simulink library "ddm"  (R2021b)
settings: Solver=VariableStepAuto  StartTime=0.0  StopTime=10.0  RelTol=1e-3
undefined symbols (not defined in the file or in its folder): ADDM_FrTMTqDev_X_Nm, ADDM_RrTMTqDev_X_Nm, ENUM_ADASACCSTA_ERROR, ENUM_ADASACCSTA_OFF, ENUM_ADASACCSTA_STANDBY, ENUM_ALLOWMOV_ALLOWREADY, ENUM_APS, ENUM_BRKSTA_ERROR, ENUM_BRKSTA_OFF, ENUM_BRKSTA_ON, ENUM_BRKSW_INVALID, ENUM_BRKSW_OFF, ENUM_BRKSW_ON, ENUM_CHGPREACTERRSTA_OBCPRE, ENUM_DCDCFAULTSTA_ANYFAULTLV1, ENUM_DCDCFAULTSTA_ANYFAULTLV2, ENUM_DRIVETRAIN_AWD, ENUM_DRIVETRAIN_FWD, ENUM_DRIVETRAIN_RWD, ENUM_EDUDRTSTA_NORMAL, ENUM_EPBSTA_APPLIED, ENUM_EPBSTA_RELEASED, ENUM_GEARACTUALPOSN_INVALID, ENUM_GEARACTUALPOSN_P, ENUM_HVBATTREADYPRE_READY, ENUM_MCUWARN_LV0, ENUM_MCUWARN_LV1, ENUM_MCUWARN_LV2, ENUM_MCUWARN_LV3, ENUM_MCUWARN_NOERROR, ENUM_OBCFAULTSTA_ANYFAULT, ENUM_PAS_R2F2, ENUM_PDFAULT_BATTPDFAIL, ENUM_PDFAULT_DCDCDISABLE, ENUM_PDFAULT_MCUDISABLE, ENUM_PDFAULT_MCUDISCHRG, ENUM_POWERSTA_OFF, ENUM_POWERSTA_ON, ENUM_POWERSTA_READY, ENUM_POWERSTA_STANDBY, ENUM_PRESSINDI_LOW, ENUM_PUFAULT_BATTUPFAIL, ENUM_PUFAULT_DCDCENABLEFAIL, ENUM_PUFAULT_PRECHRGCHKFAIL, ENUM_PUFAULT_SAFETYCHKFAIL, ENUM_PUSTATE_COMPLETED, ENUM_PWRSTASW_OFF, ENUM_PWRSTASW_OFFA, ENUM_PWRSTASW_OFFCHVCHRG, ENUM_PWRSTASW_OFFCLVCHRG, ENUM_PWRSTASW_ON, ENUM_PWRSTASW_ONHVCHRG, ENUM_PWRSTASW_READY, ENUM_PWRSTASW_STANDBY, ENUM_SHIFTCOMMAND_P, ENUM_SHIFTERERRSTA_PBUTTONFAILURE, ENUM_VEHMALFUNLV_2ND, ENUM_VEHMALFUNLV_3RD, ENUM_VEHMALFUNLV_4TH, ENUM_VEHMALFUNLV_NORMAL ... (+459)
libraries: hcu_lib x515, simulink x3
(part 17 of 25)

== system ddm/DDM/DDM/PMM/Comm err/The CAN signal between VCU and BMS1 is discontinuous ==
  note: Test Detection Criteria
  note: Test Pass Criteria
  note: Release Condition After Decision
  note: Diagnostics and Fault Handling
  task_time_s : Inport
  VPMM_PowerSta_enum : Inport  Port=2
  VPMM_PwrStaSW_enum : Inport  Port=3
  VDDM_C3BMS1RCChk_flg : Inport  Port=4
  VDDM_C3BMS1LCCFS_flg : Inport  Port=5
  No_CAN3_BUS_OFF : Inport  Port=6
  DTC_clear_request : Inport  Port=7
  Constant1 : Constant  Value=TRUE
  Constant10 : Constant  Value=ENUM_POWERSTA_STANDBY
  Constant11 : Constant  Value=ZERO_INT
  Constant12 : Constant  Value=FALSE
  Constant13 : Constant  Value=KDDM_C3BMS1RCDTC_cnt
  Constant14 : Constant  Value=KDDM_C3BMS1RCDetTO_s
  Constant17 : Constant  Value=KDDM_C3BMS1RCDTC_cnt
  Constant29 : Constant  Value=ENUM_PWRSTASW_OFF
  Constant30 : Constant  Value=KDDM_CommErrDiagnosisOffSW_flg
  Constant31 : Constant  Value=ENUM_POWERSTA_OFF
  Constant6 : Constant  Value=KDDM_C3BMS1RCPassTO_s
  Constant7 : Constant  Value=KDDM_C3BMS1RCPassTO_s
  Constant8 : Constant  Value=FALSE
  Constant9 : Constant  Value=ENUM_PWRSTASW_OFF
  DTC_Couter1 : hcu_lib/Basic_Blocks/DTC_Couter
  DTC_Info : hcu_lib/Basic_Blocks/DTC_Info
  Delay1 : Delay  DelayLength=1
  Equal1 : RelationalOperator  Operator=~=  OutDataTypeStr=boolean  RndMeth=Simplest
  Equal5 : RelationalOperator  Operator=~=  OutDataTypeStr=boolean  RndMeth=Simplest
  Equal6 : RelationalOperator  OutDataTypeStr=boolean  RndMeth=Simplest
  Equal7 : RelationalOperator  Operator===  OutDataTypeStr=boolean  RndMeth=Simplest
  Equal8 : RelationalOperator  Operator===  OutDataTypeStr=boolean  RndMeth=Simplest
  Logical Operator10 : Logic  Operator=NOT  AllPortsSameDT=off  OutDataTypeStr=boolean
  Logical Operator11 : Logic  Inputs=3  AllPortsSameDT=off  OutDataTypeStr=boolean
  Logical Operator13 : Logic  Operator=NOT  AllPortsSameDT=off  OutDataTypeStr=boolean
  Logical Operator14 : Logic  Operator=OR  Inputs=4  AllPortsSameDT=off  OutDataTypeStr=boolean
  Logical Operator16 : Logic  AllPortsSameDT=off  OutDataTypeStr=boolean
  Logical Operator17 : Logic  Inputs=3  AllPortsSameDT=off  OutDataTypeStr=boolean
  Logical Operator20 : Logic  Operator=NOT  AllPortsSameDT=off  OutDataTypeStr=boolean
  Logical Operator22 : Logic  AllPortsSameDT=off  OutDataTypeStr=boolean
  NOT1 : Logic  Operator=NOT  AllPortsSameDT=off  OutDataTypeStr=boolean
  Relational Operator1 : RelationalOperator  Operator=>  OutDataTypeStr=boolean  RndMeth=Simplest
  Switch2 : Switch  Criteria=u2 ~= 0
  Switch8 : Switch  Criteria=u2 ~= 0
  Switch9 : Switch  Criteria=u2 ~= 0
  Terminator : Terminator
  Test Detection Criteria : hcu_lib/Basic_Blocks/Test Detection Criteria
  Timer2 : hcu_lib/Basic_Blocks/Timer
  Unit Delay1 : UnitDelay  SampleTime=-1  HasFrameUpgradeWarning=on
  VDDM_C3BMS1RCDTC_raw32 : Outport
  VDDM_C3BMS1RCCFS_flg : Outport  Port=2
  wires:
  [VDDM_C3BMS1RCCFS_flg] -> VDDM_C3BMS1RCCFS_flg/1
  DTC_Couter1/2 -> Relational Operator1/1  "VDDM_C3BMS1RCDTC_cnt"
  Constant6/1 -> Timer2/4
  DTC_Couter1/1 -> [VDDM_C3BMS1RCCFS_flg]  "VDDM_C3BMS1RCCFS_flg"
  Delay1/1 -> NOT1/1
  [VDDM_C3BMS1RCDet_flg] -> DTC_Couter1/1
  Logical Operator16/1 -> Logical Operator14/1
  Unit Delay1/1 -> Equal7/1
  Equal1/1 -> Logical Operator11/2
  [DTC_clear_request] -> Logical Operator14/2
  Constant31/1 -> Equal7/2
  Equal7/1 -> Logical Operator16/1
  Test Detection Criteria/1 -> [VDDM_C3BMS1RCDet_flg]  "VDDM_C3BMS1RCDet_flg"
  [VPMM_PowerSta_enum] -> Equal8/1
  Switch9/1 -> Test Detection Criteria/1
  Constant30/1 -> Logical Operator14/4
  Constant10/1 -> Equal8/2
  [task_time_s] -> Timer2/3
  Logical Operator14/1 -> [VDDM_C3BMS1RCCFSRls_flg]  "VDDM_C3BMS1RCCFSRls_flg"
  [VDDM_C3BMS1RCChk_flg] -> Switch8/1
  [VDDM_C3BMS1RCCFS_flg] -> Delay1/1
  Constant13/1 -> Test Detection Criteria/3
  [VPMM_PowerSta_enum] -> Unit Delay1/1
  Relational Operator1/1 -> Terminator/1  "VDDM_C3BMS1RCDFS_flg"
  NOT1/1 -> Logical Operator22/2
  Constant1/1 -> Switch8/3
  Logical Operator22/1 -> Logical Operator14/3
  Equal8/1 -> Logical Operator16/2
  Constant9/1 -> Equal1/2
  Equal5/1 -> Logical Operator17/2
  [VDDM_C3BMS1RCPass_flg] -> Logical Operator22/1
  [task_time_s] -> Test Detection Criteria/2
  Switch2/1 -> Switch9/3
  Logical Operator11/1 -> Switch2/2
  [No_CAN3_BUS_OFF] -> Logical Operator11/1
  Logical Operator13/1 -> Logical Operator17/3
  Constant17/1 -> DTC_Couter1/3
  [VDDM_C3BMS1RCChk_flg] -> Switch2/1
  Equal6/1 -> [VDDM_C3BMS1RCPass_flg]  "VDDM_C3BMS1RCPass_flg"
  [VDDM_C3BMS1RCCFSRls_flg] -> Switch9/2
  [VDDM_C3BMS1LCCFS_flg] -> Logical Operator13/1
  [VPMM_PwrStaSW_enum] -> Equal1/1
  Constant8/1 -> Switch9/1
  Constant14/1 -> Test Detection Criteria/4
  Logical Operator10/1 -> Logical Operator11/3
  Constant7/1 -> Equal6/2
  [No_CAN3_BUS_OFF] -> Logical Operator17/1
  [VPMM_PwrStaSW_enum] -> Equal5/1
  Logical Operator17/1 -> Switch8/2
  [VDDM_C3BMS1LCCFS_flg] -> Logical Operator10/1
  Constant29/1 -> Equal5/2
  Switch8/1 -> Logical Operator20/1, Timer2/2
  Timer2/1 -> Equal6/1
  Constant12/1 -> Switch2/3
  Logical Operator20/1 -> Timer2/1
  [VDDM_C3BMS1RCCFSRls_flg] -> DTC_Couter1/2
  Constant11/1 -> Relational Operator1/2
  VPMM_PowerSta_enum/1 -> [VPMM_PowerSta_enum]
  VPMM_PwrStaSW_enum/1 -> [VPMM_PwrStaSW_enum]
  VDDM_C3BMS1RCChk_flg/1 -> [VDDM_C3BMS1RCChk_flg]
  task_time_s/1 -> [task_time_s]
  VDDM_C3BMS1LCCFS_flg/1 -> [VDDM_C3BMS1LCCFS_flg]
  No_CAN3_BUS_OFF/1 -> [No_CAN3_BUS_OFF]
  DTC_clear_request/1 -> [DTC_clear_request]
  [VDDM_C3BMS1RCPass_flg] -> DTC_Info/2
  [VDDM_C3BMS1RCCFS_flg] -> DTC_Info/3
  DTC_Info/1 -> VDDM_C3BMS1RCDTC_raw32/1  "VDDM_C3BMS1RCDTC_raw32"
  [VDDM_C3BMS1RCDet_flg] -> DTC_Info/1
  [DTC_clear_request] -> DTC_Info/4

== system ddm/DDM/DDM/PMM/Comm err/The CAN signal between VCU and BMS1 is incomplete ==
  note: Test Detection Criteria
  note: Release Condition After Decision
  note: Diagnostics and Fault Handling
  note: Test Pass Criteria
  task_time_s : Inport
  VPMM_PowerSta_enum : Inport  Port=2
  VPMM_PwrStaSW_enum : Inport  Port=3
  VDDM_C3BMS1CSChk_flg : Inport  Port=4
  VDDM_C3BMS1LCCFS_flg : Inport  Port=5
  No_CAN3_BUS_OFF : Inport  Port=6
  DTC_clear_request : Inport  Port=7
  Constant1 : Constant  Value=KDDM_C3BMS1CSDTC_cnt
  Constant10 : Constant  Value=ENUM_POWERSTA_STANDBY
  Constant11 : Constant  Value=ZERO_INT
  Constant12 : Constant  Value=ENUM_PWRSTASW_OFF
  Constant13 : Constant  Value=FALSE
  Constant14 : Constant  Value=KDDM_C3BMS1CSPassTO_s
  Constant29 : Constant  Value=ENUM_PWRSTASW_OFF
  Constant30 : Constant  Value=KDDM_CommErrDiagnosisOffSW_flg
  Constant31 : Constant  Value=ENUM_POWERSTA_OFF
  Constant32 : Constant  Value=KDDM_C3BMS1CSDTC_cnt
  Constant33 : Constant  Value=KDDM_C3BMS1CSDetTO_s
  Constant6 : Constant  Value=TRUE
  Constant7 : Constant  Value=KDDM_C3BMS1CSPassTO_s
  Constant9 : Constant  Value=FALSE
  DTC_Couter1 : hcu_lib/Basic_Blocks/DTC_Couter
  DTC_Info : hcu_lib/Basic_Blocks/DTC_Info
  Delay1 : Delay  DelayLength=1
  Equal1 : RelationalOperator  Operator=~=  OutDataTypeStr=boolean  RndMeth=Simplest
  Equal5 : RelationalOperator  Operator=~=  OutDataTypeStr=boolean  RndMeth=Simplest
  Equal6 : RelationalOperator  OutDataTypeStr=boolean  RndMeth=Simplest
  Equal7 : RelationalOperator  Operator===  OutDataTypeStr=boolean  RndMeth=Simplest
  Equal8 : RelationalOperator  Operator===  OutDataTypeStr=boolean  RndMeth=Simplest
  Logical Operator10 : Logic  Operator=NOT  AllPortsSameDT=off  OutDataTypeStr=boolean
  Logical Operator11 : Logic  Inputs=3  AllPortsSameDT=off  OutDataTypeStr=boolean
  Logical Operator13 : Logic  Operator=NOT  AllPortsSameDT=off  OutDataTypeStr=boolean
  Logical Operator14 : Logic  Operator=OR  Inputs=4  AllPortsSameDT=off  OutDataTypeStr=boolean
  Logical Operator16 : Logic  AllPortsSameDT=off  OutDataTypeStr=boolean
  Logical Operator17 : Logic  Inputs=3  AllPortsSameDT=off  OutDataTypeStr=boolean
  Logical Operator20 : Logic  Operator=NOT  AllPortsSameDT=off  OutDataTypeStr=boolean
  Logical Operator22 : Logic  AllPortsSameDT=off  OutDataTypeStr=boolean
  NOT1 : Logic  Operator=NOT  AllPortsSameDT=off  OutDataTypeStr=boolean
  Relational Operator1 : RelationalOperator  Operator=>  OutDataTypeStr=boolean  RndMeth=Simplest
  Switch2 : Switch  Criteria=u2 ~= 0
  Switch8 : Switch  Criteria=u2 ~= 0
  Switch9 : Switch  Criteria=u2 ~= 0
  Terminator : Terminator
  Test Detection Criteria1 : hcu_lib/Basic_Blocks/Test Detection Criteria
  Timer2 : hcu_lib/Basic_Blocks/Timer
  Unit Delay1 : UnitDelay  SampleTime=-1  HasFrameUpgradeWarning=on
  VDDM_C3BMS1CSDTC_raw32 : Outport
  VDDM_C3BMS1CSCFS_flg : Outport  Port=2
  wires:
  [VDDM_C3BMS1CSCFS_flg] -> VDDM_C3BMS1CSCFS_flg/1
  [task_time_s] -> Timer2/3
  Timer2/1 -> Equal6/1
  [VDDM_C3BMS1LCCFS_flg] -> Logical Operator10/1
  Constant29/1 -> Equal5/2
  [VDDM_C3BMS1CSChk_flg] -> Switch2/1
  Logical Operator20/1 -> Timer2/1
  Logical Operator16/1 -> Logical Operator14/1
  Relational Operator1/1 -> Terminator/1  "VDDM_C3BMS1CSDFS_flg"
  Constant1/1 -> DTC_Couter1/3
  Test Detection Criteria1/1 -> [VDDM_C3BMS1CSDet_flg]  "VDDM_C3BMS1CSDet_flg"
  Constant12/1 -> Equal1/2
  [VDDM_C3BMS1CSChk_flg] -> Switch8/1
  [VDDM_C3BMS1CSCFS_flg] -> Delay1/1
  Equal7/1 -> Logical Operator16/1
  Equal6/1 -> [VDDM_C3BMS1CSPass_flg]  "VDDM_C3BMS1CSPass_flg"
  [VPMM_PowerSta_enum] -> Unit Delay1/1
  [VDDM_C3BMS1CSDet_flg] -> DTC_Couter1/1
  [No_CAN3_BUS_OFF] -> Logical Operator17/1
  DTC_Couter1/1 -> [VDDM_C3BMS1CSCFS_flg]  "VDDM_C3BMS1CSCFS_flg"
  [VPMM_PwrStaSW_enum] -> Equal1/1
  Constant31/1 -> Equal7/2
  [VDDM_C3BMS1CSPass_flg] -> Logical Operator22/1
  Constant33/1 -> Test Detection Criteria1/4
  Constant32/1 -> Test Detection Criteria1/3
  Unit Delay1/1 -> Equal7/1
  Switch8/1 -> Logical Operator20/1, Timer2/2
  Equal1/1 -> Logical Operator11/2
  [DTC_clear_request] -> Logical Operator14/2
  Constant14/1 -> Timer2/4
  [VDDM_C3BMS1CSCFSRls_flg] -> DTC_Couter1/2
  Delay1/1 -> NOT1/1
  DTC_Couter1/2 -> Relational Operator1/1  "VDDM_C3BMS1CSDTC_cnt"
  Constant11/1 -> Relational Operator1/2
  [VDDM_C3BMS1LCCFS_flg] -> Logical Operator13/1
  Constant13/1 -> Switch2/3
  Logical Operator10/1 -> Logical Operator11/3
  Logical Operator17/1 -> Switch8/2
  [VPMM_PwrStaSW_enum] -> Equal5/1
  Constant10/1 -> Equal8/2
  Logical Operator13/1 -> Logical Operator17/3
  Constant9/1 -> Switch9/1
  [No_CAN3_BUS_OFF] -> Logical Operator11/1
  Switch2/1 -> Switch9/3
  [task_time_s] -> Test Detection Criteria1/2
  [VPMM_PowerSta_enum] -> Equal8/1
  Equal8/1 -> Logical Operator16/2
  Equal5/1 -> Logical Operator17/2
  Logical Operator11/1 -> Switch2/2
  NOT1/1 -> Logical Operator22/2
  Logical Operator22/1 -> Logical Operator14/3
  Constant6/1 -> Switch8/3
  Constant30/1 -> Logical Operator14/4
  Switch9/1 -> Test Detection Criteria1/1
  Logical Operator14/1 -> [VDDM_C3BMS1CSCFSRls_flg]  "VDDM_C3BMS1CSCFSRls_flg"
  Constant7/1 -> Equal6/2
  [VDDM_C3BMS1CSCFSRls_flg] -> Switch9/2
  task_time_s/1 -> [task_time_s]
  VDDM_C3BMS1CSChk_flg/1 -> [VDDM_C3BMS1CSChk_flg]
  VPMM_PwrStaSW_enum/1 -> [VPMM_PwrStaSW_enum]
  VPMM_PowerSta_enum/1 -> [VPMM_PowerSta_enum]
  VDDM_C3BMS1LCCFS_flg/1 -> [VDDM_C3BMS1LCCFS_flg]
  No_CAN3_BUS_OFF/1 -> [No_CAN3_BUS_OFF]
  DTC_clear_request/1 -> [DTC_clear_request]
  DTC_Info/1 -> VDDM_C3BMS1CSDTC_raw32/1  "VDDM_C3BMS1CSDTC_raw32"
  [VDDM_C3BMS1CSCFS_flg] -> DTC_Info/3
  [VDDM_C3BMS1CSDet_flg] -> DTC_Info/1
  [VDDM_C3BMS1CSPass_flg] -> DTC_Info/2
  [DTC_clear_request] -> DTC_Info/4

== system ddm/DDM/DDM/PMM/Comm err/The CAN signal between VCU and BMS6 is discontinuous ==
  note: Test Detection Criteria
  note: Test Pass Criteria
  note: Release Condition After Decision
  note: Diagnostics and Fault Handling
  task_time_s : Inport
  VPMM_PowerSta_enum : Inport  Port=2
  VPMM_PwrStaSW_enum : Inport  Port=3
  VDDM_C3BMS6RCChk_flg : Inport  Port=4
  VDDM_C3BMS6LCCFS_flg : Inport  Port=5
  No_CAN3_BUS_OFF : Inport  Port=6
  DTC_clear_request : Inport  Port=7
  Constant10 : Constant  Value=ENUM_POWERSTA_STANDBY
  Constant11 : Constant  Value=ZERO_INT
  Constant16 : Constant  Value=TRUE
  Constant18 : Constant  Value=KDDM_C3BMS6RCPassTO_s
  Constant19 : Constant  Value=KDDM_C3BMS6RCPassTO_s
  Constant2 : Constant  Value=FALSE
  Constant3 : Constant  Value=ENUM_PWRSTASW_OFF
  Constant4 : Constant  Value=FALSE
  Constant40 : Constant  Value=KDDM_C3BMS6RCDTC_cnt
  Constant41 : Constant  Value=KDDM_C3BMS6RCDetTO_s
  Constant48 : Constant  Value=KDDM_C3BMS6RCDTC_cnt
  Constant5 : Constant  Value=ENUM_PWRSTASW_OFF
  Constant7 : Constant  Value=KDDM_CommErrDiagnosisOffSW_flg
  Constant8 : Constant  Value=ENUM_POWERSTA_OFF
  DTC_Couter : hcu_lib/Basic_Blocks/DTC_Couter
  DTC_Info : hcu_lib/Basic_Blocks/DTC_Info
  Delay1 : Delay  DelayLength=1
  Equal : RelationalOperator  Operator=~=  OutDataTypeStr=boolean  RndMeth=Simplest
  Equal2 : RelationalOperator  Operator=~=  OutDataTypeStr=boolean  RndMeth=Simplest
  Equal3 : RelationalOperator  OutDataTypeStr=boolean  RndMeth=Simplest
  Equal4 : RelationalOperator  Operator===  OutDataTypeStr=boolean  RndMeth=Simplest
  Equal6 : RelationalOperator  Operator===  OutDataTypeStr=boolean  RndMeth=Simplest
  Logical Operator1 : Logic  Operator=NOT  AllPortsSameDT=off  OutDataTypeStr=boolean
  Logical Operator14 : Logic  Operator=OR  Inputs=4  AllPortsSameDT=off  OutDataTypeStr=boolean
  Logical Operator16 : Logic  AllPortsSameDT=off  OutDataTypeStr=boolean
  Logical Operator2 : Logic  Inputs=3  AllPortsSameDT=off  OutDataTypeStr=boolean
  Logical Operator4 : Logic  Operator=NOT  AllPortsSameDT=off  OutDataTypeStr=boolean
  Logical Operator5 : Logic  Inputs=3  AllPortsSameDT=off  OutDataTypeStr=boolean
  Logical Operator6 : Logic  Operator=NOT  AllPortsSameDT=off  OutDataTypeStr=boolean
  Logical Operator8 : Logic  AllPortsSameDT=off  OutDataTypeStr=boolean
  NOT1 : Logic  Operator=NOT  AllPortsSameDT=off  OutDataTypeStr=boolean
  Relational Operator1 : RelationalOperator  Operator=>  OutDataTypeStr=boolean  RndMeth=Simplest
  Switch3 : Switch  Criteria=u2 ~= 0
  Switch4 : Switch  Criteria=u2 ~= 0
  Switch6 : Switch  Criteria=u2 ~= 0
  Terminator : Terminator
  Test Detection Criteria : hcu_lib/Basic_Blocks/Test Detection Criteria
  Timer1 : hcu_lib/Basic_Blocks/Timer
  Unit Delay1 : UnitDelay  SampleTime=-1  HasFrameUpgradeWarning=on
  VDDM_C3BMS6RCDTC_raw32 : Outport
  VDDM_C3BMS6RCCFS_flg : Outport  Port=2
  wires:
  Relational Operator1/1 -> Terminator/1  "VDDM_C3BMS6RCDFS_flg"
  Constant11/1 -> Relational Operator1/2
  [VDDM_C3BMS6RCCFSRls_flg] -> DTC_Couter/2
  Delay1/1 -> NOT1/1
  [VDDM_C3BMS6RCPass_flg] -> Logical Operator8/1
  Equal6/1 -> Logical Operator16/2
  Logical Operator8/1 -> Logical Operator14/3
  Logical Operator14/1 -> [VDDM_C3BMS6RCCFSRls_flg]  "VDDM_C3BMS6RCCFSRls_flg"
  Constant10/1 -> Equal6/2
  [VDDM_C3BMS6RCCFS_flg] -> Delay1/1
  NOT1/1 -> Logical Operator8/2
  Constant7/1 -> Logical Operator14/4
  [VPMM_PowerSta_enum] -> Unit Delay1/1
  Constant8/1 -> Equal4/2
  Equal4/1 -> Logical Operator16/1
  Logical Operator16/1 -> Logical Operator14/1
  [VPMM_PowerSta_enum] -> Equal6/1
  Unit Delay1/1 -> Equal4/1
  [DTC_clear_request] -> Logical Operator14/2
  task_time_s/1 -> [task_time_s]
  VDDM_C3BMS6RCChk_flg/1 -> [VDDM_C3BMS6RCChk_flg]
  VPMM_PwrStaSW_enum/1 -> [VPMM_PwrStaSW_enum]
  VPMM_PowerSta_enum/1 -> [VPMM_PowerSta_enum]
  No_CAN3_BUS_OFF/1 -> [No_CAN3_BUS_OFF]
  Logical Operator2/1 -> Switch3/2
  [task_time_s] -> Test Detection Criteria/2
  Constant40/1 -> Test Detection Criteria/3
  Switch3/1 -> Switch6/3
  Constant3/1 -> Equal/2
  Constant4/1 -> Switch3/3
  [VDDM_C3BMS6RCChk_flg] -> Switch3/1
  Equal/1 -> Logical Operator2/2
  [No_CAN3_BUS_OFF] -> Logical Operator2/1
  Constant5/1 -> Equal2/2
  Equal3/1 -> [VDDM_C3BMS6RCPass_flg]  "VDDM_C3BMS6RCPass_flg"
  Logical Operator6/1 -> Timer1/1
  Logical Operator5/1 -> Switch4/2
  Constant19/1 -> Equal3/2
  Switch4/1 -> Logical Operator6/1, Timer1/2
  [VDDM_C3BMS6RCChk_flg] -> Switch4/1
  Timer1/1 -> Equal3/1
  [No_CAN3_BUS_OFF] -> Logical Operator5/1
  Constant18/1 -> Timer1/4
  Equal2/1 -> Logical Operator5/2
  Constant16/1 -> Switch4/3
  DTC_clear_request/1 -> [DTC_clear_request]
  VDDM_C3BMS6LCCFS_flg/1 -> [VDDM_C3BMS6LCCFS_flg]
  [VDDM_C3BMS6LCCFS_flg] -> Logical Operator1/1
  Logical Operator1/1 -> Logical Operator2/3
  [VDDM_C3BMS6LCCFS_flg] -> Logical Operator4/1
  Logical Operator4/1 -> Logical Operator5/3
  [VPMM_PwrStaSW_enum] -> Equal/1
  [VPMM_PwrStaSW_enum] -> Equal2/1
  [task_time_s] -> Timer1/3
  [VDDM_C3BMS6RCCFS_flg] -> DTC_Info/3
  DTC_Info/1 -> VDDM_C3BMS6RCDTC_raw32/1  "VDDM_C3BMS6RCDTC_raw32"
  Test Detection Criteria/1 -> [VDDM_C3BMS6RCDet_flg]  "VDDM_C3BMS6RCDet_flg"
  Constant41/1 -> Test Detection Criteria/4
  [VDDM_C3BMS6RCDet_flg] -> DTC_Info/1
  [VDDM_C3BMS6RCPass_flg] -> DTC_Info/2
  [DTC_clear_request] -> DTC_Info/4
  Constant2/1 -> Switch6/1
  Switch6/1 -> Test Detection Criteria/1
  [VDDM_C3BMS6RCCFSRls_flg] -> Switch6/2
  [VDDM_C3BMS6RCCFS_flg] -> VDDM_C3BMS6RCCFS_flg/1
  Constant48/1 -> DTC_Couter/3
  DTC_Couter/1 -> [VDDM_C3BMS6RCCFS_flg]  "VDDM_C3BMS6RCCFS_flg"
  [VDDM_C3BMS6RCDet_flg] -> DTC_Couter/1
  DTC_Couter/2 -> Relational Operator1/1  "VDDM_C3BMS6RCDTC_cnt"

== system ddm/DDM/DDM/PMM/Comm err/The CAN signal between VCU and BMS6 is incomplete ==
  note: Test Detection Criteria
  note: Test Pass Criteria
  note: Release Condition After Decision
  note: Diagnostics and Fault Handling
  task_time_s : Inport
  VPMM_PowerSta_enum : Inport  Port=2
  VPMM_PwrStaSW_enum : Inport  Port=3
  VDDM_C3BMS6CSChk_flg : Inport  Port=4
  VDDM_C3BMS6LCCFS_flg : Inport  Port=5
  No_CAN3_BUS_OFF : Inport  Port=6
  DTC_clear_request : Inport  Port=7
  Constant10 : Constant  Value=ENUM_POWERSTA_STANDBY
  Constant11 : Constant  Value=ZERO_INT
  Constant12 : Constant  Value=ENUM_PWRSTASW_OFF
  Constant13 : Constant  Value=FALSE
  Constant14 : Constant  Value=KDDM_C3BMS6CSPassTO_s
  Constant27 : Constant  Value=KDDM_C3BMS6CSDTC_cnt
  Constant29 : Constant  Value=ENUM_PWRSTASW_OFF
  Constant30 : Constant  Value=KDDM_CommErrDiagnosisOffSW_flg
  Constant31 : Constant  Value=ENUM_POWERSTA_OFF
  Constant32 : Constant  Value=KDDM_C3BMS6CSDTC_cnt
  Constant33 : Constant  Value=KDDM_C3BMS6CSDetTO_s
  Constant6 : Constant  Value=TRUE
  Constant7 : Constant  Value=KDDM_C3BMS6CSPassTO_s
  Constant9 : Constant  Value=FALSE
  DTC_Couter1 : hcu_lib/Basic_Blocks/DTC_Couter
  DTC_Info : hcu_lib/Basic_Blocks/DTC_Info
  Delay1 : Delay  DelayLength=1
  Equal2 : RelationalOperator  Operator=~=  OutDataTypeStr=boolean  RndMeth=Simplest
  Equal5 : RelationalOperator  Operator=~=  OutDataTypeStr=boolean  RndMeth=Simplest
  Equal6 : RelationalOperator  OutDataTypeStr=boolean  RndMeth=Simplest
  Equal7 : RelationalOperator  Operator===  OutDataTypeStr=boolean  RndMeth=Simplest
  Equal8 : RelationalOperator  Operator===  OutDataTypeStr=boolean  RndMeth=Simplest
  Logical Operator10 : Logic  Operator=NOT  AllPortsSameDT=off  OutDataTypeStr=boolean
  Logical Operator11 : Logic  Inputs=3  AllPortsSameDT=off  OutDataTypeStr=boolean
  Logical Operator13 : Logic  Operator=NOT  AllPortsSameDT=off  OutDataTypeStr=boolean
  Logical Operator14 : Logic  Operator=OR  Inputs=4  AllPortsSameDT=off  OutDataTypeStr=boolean
  Logical Operator16 : Logic  AllPortsSameDT=off  OutDataTypeStr=boolean
  Logical Operator17 : Logic  Inputs=3  AllPortsSameDT=off  OutDataTypeStr=boolean
  Logical Operator20 : Logic  Operator=NOT  AllPortsSameDT=off  OutDataTypeStr=boolean
  Logical Operator22 : Logic  AllPortsSameDT=off  OutDataTypeStr=boolean
  NOT1 : Logic  Operator=NOT  AllPortsSameDT=off  OutDataTypeStr=boolean
  Relational Operator1 : RelationalOperator  Operator=>  OutDataTypeStr=boolean  RndMeth=Simplest
  Switch2 : Switch  Criteria=u2 ~= 0
  Switch8 : Switch  Criteria=u2 ~= 0
  Switch9 : Switch  Criteria=u2 ~= 0
  Terminator : Terminator
  Test Detection Criteria1 : hcu_lib/Basic_Blocks/Test Detection Criteria
  Timer2 : hcu_lib/Basic_Blocks/Timer
  Unit Delay1 : UnitDelay  SampleTime=-1  HasFrameUpgradeWarning=on
  VDDM_C3BMS6CSDTC_raw32 : Outport
  VDDM_C3BMS6CSCFS_flg : Outport  Port=2
  wires:
  Test Detection Criteria1/1 -> [VDDM_C3BMS6CSDet_flg]  "VDDM_C3BMS6CSDet_flg"
  DTC_Couter1/2 -> Relational Operator1/1  "VDDM_C3BMS6CSDTC_cnt"
  Constant14/1 -> Timer2/4
  DTC_Couter1/1 -> [VDDM_C3BMS6CSCFS_flg]  "VDDM_C3BMS6CSCFS_flg"
  Delay1/1 -> NOT1/1
  [VDDM_C3BMS6CSDet_flg] -> DTC_Couter1/1
  Logical Operator16/1 -> Logical Operator14/1
  Unit Delay1/1 -> Equal7/1
  Equal2/1 -> Logical Operator11/2
  [DTC_clear_request] -> Logical Operator14/2
  Constant31/1 -> Equal7/2
  Equal7/1 -> Logical Operator16/1
  [VPMM_PowerSta_enum] -> Equal8/1
  Switch9/1 -> Test Detection Criteria1/1
  Constant30/1 -> Logical Operator14/4
  Constant10/1 -> Equal8/2
  [task_time_s] -> Timer2/3
  Logical Operator14/1 -> [VDDM_C3BMS6CSCFSRls_flg]  "VDDM_C3BMS6CSCFSRls_flg"
  [VDDM_C3BMS6CSChk_flg] -> Switch8/1
  [VDDM_C3BMS6CSCFS_flg] -> Delay1/1
  Constant32/1 -> Test Detection Criteria1/3
  [VPMM_PowerSta_enum] -> Unit Delay1/1
  Relational Operator1/1 -> Terminator/1  "VDDM_C3BMS6CSDFS_flg"
  NOT1/1 -> Logical Operator22/2
  Constant6/1 -> Switch8/3
  Logical Operator22/1 -> Logical Operator14/3
  Equal8/1 -> Logical Operator16/2
  Constant12/1 -> Equal2/2
  Equal5/1 -> Logical Operator17/2
  [VDDM_C3BMS6CSPass_flg] -> Logical Operator22/1
  [task_time_s] -> Test Detection Criteria1/2
  Switch2/1 -> Switch9/3
  Logical Operator11/1 -> Switch2/2
  [No_CAN3_BUS_OFF] -> Logical Operator11/1
  Logical Operator13/1 -> Logical Operator17/3
  Constant27/1 -> DTC_Couter1/3
  [VDDM_C3BMS6CSChk_flg] -> Switch2/1
  Equal6/1 -> [VDDM_C3BMS6CSPass_flg]  "VDDM_C3BMS6CSPass_flg"
  [VDDM_C3BMS6CSCFSRls_flg] -> Switch9/2
  [VDDM_C3BMS6LCCFS_flg] -> Logical Operator13/1
  [VPMM_PwrStaSW_enum] -> Equal2/1
  Constant9/1 -> Switch9/1
  Constant33/1 -> Test Detection Criteria1/4
  Logical Operator10/1 -> Logical Operator11/3
  Constant7/1 -> Equal6/2
  [No_CAN3_BUS_OFF] -> Logical Operator17/1
  [VPMM_PwrStaSW_enum] -> Equal5/1
  Logical Operator17/1 -> Switch8/2
  [VDDM_C3BMS6LCCFS_flg] -> Logical Operator10/1
  Constant29/1 -> Equal5/2
  Switch8/1 -> Logical Operator20/1, Timer2/2
  Timer2/1 -> Equal6/1
  Constant13/1 -> Switch2/3
  Logical Operator20/1 -> Timer2/1
  [VDDM_C3BMS6CSCFSRls_flg] -> DTC_Couter1/2
  Constant11/1 -> Relational Operator1/2
  No_CAN3_BUS_OFF/1 -> [No_CAN3_BUS_OFF]
  VPMM_PowerSta_enum/1 -> [VPMM_PowerSta_enum]
  VPMM_PwrStaSW_enum/1 -> [VPMM_PwrStaSW_enum]
  VDDM_C3BMS6CSChk_flg/1 -> [VDDM_C3BMS6CSChk_flg]
  task_time_s/1 -> [task_time_s]
  DTC_clear_request/1 -> [DTC_clear_request]
  VDDM_C3BMS6LCCFS_flg/1 -> [VDDM_C3BMS6LCCFS_flg]
  [VDDM_C3BMS6CSPass_flg] -> DTC_Info/2
  [VDDM_C3BMS6CSCFS_flg] -> DTC_Info/3
  DTC_Info/1 -> VDDM_C3BMS6CSDTC_raw32/1  "VDDM_C3BMS6CSDTC_raw32"
  [VDDM_C3BMS6CSDet_flg] -> DTC_Info/1
  [DTC_clear_request] -> DTC_Info/4
  [VDDM_C3BMS6CSCFS_flg] -> VDDM_C3BMS6CSCFS_flg/1

== system ddm/DDM/DDM/PMM/Comm err/The CAN signal between VCU and CCU1 is discontinuous ==
  note: Test Detection Criteria
  note: Diagnostics and Fault Handling
  note: Release Condition After Decision
  note: Test Pass Criteria
  task_time_s : Inport
  VPMM_PowerSta_enum : Inport  Port=2
  VPMM_PwrStaSW_enum : Inport  Port=3
  VDDM_C3CCU1RCChk_flg : Inport  Port=4
  VDDM_C3CCU1LCCFS_flg : Inport  Port=5
  No_CAN3_BUS_OFF : Inport  Port=6
  DTC_clear_request : Inport  Port=7
  Constant1 : Constant  Value=TRUE
  Constant10 : Constant  Value=ENUM_POWERSTA_STANDBY
  Constant11 : Constant  Value=ZERO_INT
  Constant12 : Constant  Value=FALSE
  Constant13 : Constant  Value=KDDM_C3CCU1RCPassTO_s
  Constant29 : Constant  Value=ENUM_PWRSTASW_OFF
  Constant30 : Constant  Value=KDDM_CommErrDiagnosisOffSW_flg
  Constant31 : Constant  Value=ENUM_POWERSTA_OFF
  Constant32 : Constant  Value=KDDM_C3CCU1RCDTC_cnt
  Constant33 : Constant  Value=KDDM_C3CCU1RCDetTO_s
  Constant6 : Constant  Value=KDDM_C3CCU1RCPassTO_s
  Constant7 : Constant  Value=KDDM_C3CCU1RCDTC_cnt
  Constant8 : Constant  Value=FALSE
  Constant9 : Constant  Value=ENUM_PWRSTASW_OFF
  DTC_Couter1 : hcu_lib/Basic_Blocks/DTC_Couter
  DTC_Info : hcu_lib/Basic_Blocks/DTC_Info
  Delay1 : Delay  DelayLength=1
  Equal1 : RelationalOperator  Operator=~=  OutDataTypeStr=boolean  RndMeth=Simplest
  Equal5 : RelationalOperator  Operator=~=  OutDataTypeStr=boolean  RndMeth=Simplest
  Equal6 : RelationalOperator  OutDataTypeStr=boolean  RndMeth=Simplest
  Equal7 : RelationalOperator  Operator===  OutDataTypeStr=boolean  RndMeth=Simplest
  Equal8 : RelationalOperator  Operator===  OutDataTypeStr=boolean  RndMeth=Simplest
  Logical Operator10 : Logic  Operator=NOT  AllPortsSameDT=off  OutDataTypeStr=boolean
  Logical Operator11 : Logic  Inputs=3  AllPortsSameDT=off  OutDataTypeStr=boolean
  Logical Operator13 : Logic  Operator=NOT  AllPortsSameDT=off  OutDataTypeStr=boolean
  Logical Operator14 : Logic  Operator=OR  Inputs=4  AllPortsSameDT=off  OutDataTypeStr=boolean
  Logical Operator16 : Logic  AllPortsSameDT=off  OutDataTypeStr=boolean
  Logical Operator17 : Logic  Inputs=3  AllPortsSameDT=off  OutDataTypeStr=boolean
  Logical Operator20 : Logic  Operator=NOT  AllPortsSameDT=off  OutDataTypeStr=boolean
  Logical Operator22 : Logic  AllPortsSameDT=off  OutDataTypeStr=boolean
  NOT1 : Logic  Operator=NOT  AllPortsSameDT=off  OutDataTypeStr=boolean
  Relational Operator1 : RelationalOperator  Operator=>  OutDataTypeStr=boolean  RndMeth=Simplest
  Switch2 : Switch  Criteria=u2 ~= 0
  Switch8 : Switch  Criteria=u2 ~= 0
  Switch9 : Switch  Criteria=u2 ~= 0
  Terminator : Terminator
  Test Detection Criteria1 : hcu_lib/Basic_Blocks/Test Detection Criteria
  Timer2 : hcu_lib/Basic_Blocks/Timer
  Unit Delay1 : UnitDelay  SampleTime=-1  HasFrameUpgradeWarning=on
  VDDM_C3CCU1RCDTC_raw32 : Outport
  VDDM_C3CCU1RCCFS_flg : Outport  Port=2
  wires:
  [DTC_clear_request] -> DTC_Info/4
  [VDDM_C3CCU1RCDet_flg] -> DTC_Info/1
  [VDDM_C3CCU1RCPass_flg] -> DTC_Info/2
  [VDDM_C3CCU1RCCFS_flg] -> DTC_Info/3
  DTC_Info/1 -> VDDM_C3CCU1RCDTC_raw32/1  "VDDM_C3CCU1RCDTC_raw32"
  DTC_clear_request/1 -> [DTC_clear_request]
  No_CAN3_BUS_OFF/1 -> [No_CAN3_BUS_OFF]
  VDDM_C3CCU1LCCFS_flg/1 -> [VDDM_C3CCU1LCCFS_flg]
  VPMM_PowerSta_enum/1 -> [VPMM_PowerSta_enum]
  VPMM_PwrStaSW_enum/1 -> [VPMM_PwrStaSW_enum]
  VDDM_C3CCU1RCChk_flg/1 -> [VDDM_C3CCU1RCChk_flg]
  task_time_s/1 -> [task_time_s]
  Equal6/1 -> [VDDM_C3CCU1RCPass_flg]  "VDDM_C3CCU1RCPass_flg"
  [No_CAN3_BUS_OFF] -> Logical Operator17/1
  Constant33/1 -> Test Detection Criteria1/4
  Constant29/1 -> Equal5/2
  Logical Operator10/1 -> Logical Operator11/3
  Timer2/1 -> Equal6/1
  Logical Operator17/1 -> Switch8/2
  Switch8/1 -> Timer2/2, Logical Operator20/1
  Constant11/1 -> Relational Operator1/2
  Constant8/1 -> Switch9/1
  Constant12/1 -> Switch2/3
  [VDDM_C3CCU1LCCFS_flg] -> Logical Operator13/1
  DTC_Couter1/2 -> Relational Operator1/1  "VDDM_C3CCU1RCDTC_cnt"
  DTC_Couter1/1 -> [VDDM_C3CCU1RCCFS_flg]  "VDDM_C3CCU1RCCFS_flg"
  Constant13/1 -> Timer2/4
  Constant31/1 -> Equal7/2
  Logical Operator20/1 -> Timer2/1
  Logical Operator16/1 -> Logical Operator14/1
  Equal1/1 -> Logical Operator11/2
  Delay1/1 -> NOT1/1
  Unit Delay1/1 -> Equal7/1
  [VDDM_C3CCU1RCCFS_flg] -> Delay1/1
  [task_time_s] -> Timer2/3
  Test Detection Criteria1/1 -> [VDDM_C3CCU1RCDet_flg]  "VDDM_C3CCU1RCDet_flg"
  [VPMM_PowerSta_enum] -> Equal8/1
  Switch9/1 -> Test Detection Criteria1/1
  Constant30/1 -> Logical Operator14/4
  Constant32/1 -> Test Detection Criteria1/3
  Constant10/1 -> Equal8/2
  [VPMM_PowerSta_enum] -> Unit Delay1/1
  [DTC_clear_request] -> Logical Operator14/2
  Constant1/1 -> Switch8/3
  Relational Operator1/1 -> Terminator/1  "VDDM_C3CCU1RCDFS_flg"
  NOT1/1 -> Logical Operator22/2
  Logical Operator22/1 -> Logical Operator14/3
  Switch2/1 -> Switch9/3
  [VPMM_PwrStaSW_enum] -> Equal5/1
  Logical Operator11/1 -> Switch2/2
  Logical Operator14/1 -> [VDDM_C3CCU1RCCFSRls_flg]  "VDDM_C3CCU1RCCFSRls_flg"
  Equal8/1 -> Logical Operator16/2
  [task_time_s] -> Test Detection Criteria1/2
  Constant9/1 -> Equal1/2
  Constant7/1 -> DTC_Couter1/3
  [VDDM_C3CCU1RCDet_flg] -> DTC_Couter1/1
  [VDDM_C3CCU1RCPass_flg] -> Logical Operator22/1
  Constant6/1 -> Equal6/2
  Logical Operator13/1 -> Logical Operator17/3
  [VDDM_C3CCU1RCChk_flg] -> Switch2/1
  Equal7/1 -> Logical Operator16/1
  Equal5/1 -> Logical Operator17/2
  [VDDM_C3CCU1RCCFSRls_flg] -> DTC_Couter1/2
  [VDDM_C3CCU1RCChk_flg] -> Switch8/1
  [VDDM_C3CCU1RCCFSRls_flg] -> Switch9/2
  [No_CAN3_BUS_OFF] -> Logical Operator11/1
  [VPMM_PwrStaSW_enum] -> Equal1/1
  [VDDM_C3CCU1LCCFS_flg] -> Logical Operator10/1
  [VDDM_C3CCU1RCCFS_flg] -> VDDM_C3CCU1RCCFS_flg/1

== system ddm/DDM/DDM/PMM/Comm err/The CAN signal between VCU and CCU1 is incomplete ==
  note: Release Condition After Decision
  note: Test Detection Criteria
  note: Test Pass Criteria
  note: Diagnostics and Fault Handling
  task_time_s : Inport
  VPMM_PowerSta_enum : Inport  Port=2
  VPMM_PwrStaSW_enum : Inport  Port=3
  VDDM_C3CCU1CSChk_flg : Inport  Port=4
  VDDM_C3CCU1LCCFS_flg : Inport  Port=5
  No_CAN3_BUS_OFF : Inport  Port=6
  DTC_clear_request : Inport  Port=7
  Constant1 : Constant  Value=KDDM_C3CCU1CSDTC_cnt
  Constant10 : Constant  Value=ENUM_POWERSTA_STANDBY
  Constant11 : Constant  Value=ZERO_INT
  Constant12 : Constant  Value=ENUM_PWRSTASW_OFF
  Constant13 : Constant  Value=FALSE
  Constant14 : Constant  Value=KDDM_C3CCU1CSPassTO_s
  Constant17 : Constant  Value=KDDM_C3CCU1CSDetTO_s
  Constant29 : Constant  Value=ENUM_PWRSTASW_OFF
  Constant30 : Constant  Value=KDDM_CommErrDiagnosisOffSW_flg
  Constant31 : Constant  Value=ENUM_POWERSTA_OFF
  Constant6 : Constant  Value=TRUE
  Constant7 : Constant  Value=KDDM_C3CCU1CSPassTO_s
  Constant8 : Constant  Value=KDDM_C3CCU1CSDTC_cnt
  Constant9 : Constant  Value=FALSE
  DTC_Couter1 : hcu_lib/Basic_Blocks/DTC_Couter
  DTC_Info : hcu_lib/Basic_Blocks/DTC_Info
  Delay1 : Delay  DelayLength=1
  Equal1 : RelationalOperator  Operator=~=  OutDataTypeStr=boolean  RndMeth=Simplest
  Equal5 : RelationalOperator  Operator=~=  OutDataTypeStr=boolean  RndMeth=Simplest
  Equal6 : RelationalOperator  OutDataTypeStr=boolean  RndMeth=Simplest
  Equal7 : RelationalOperator  Operator===  OutDataTypeStr=boolean  RndMeth=Simplest
  Equal8 : RelationalOperator  Operator===  OutDataTypeStr=boolean  RndMeth=Simplest
  Logical Operator10 : Logic  Operator=NOT  AllPortsSameDT=off  OutDataTypeStr=boolean
  Logical Operator11 : Logic  Inputs=3  AllPortsSameDT=off  OutDataTypeStr=boolean
  Logical Operator13 : Logic  Operator=NOT  AllPortsSameDT=off  OutDataTypeStr=boolean
  Logical Operator14 : Logic  Operator=OR  Inputs=4  AllPortsSameDT=off  OutDataTypeStr=boolean
  Logical Operator16 : Logic  AllPortsSameDT=off  OutDataTypeStr=boolean
  Logical Operator17 : Logic  Inputs=3  AllPortsSameDT=off  OutDataTypeStr=boolean
  Logical Operator20 : Logic  Operator=NOT  AllPortsSameDT=off  OutDataTypeStr=boolean
  Logical Operator22 : Logic  AllPortsSameDT=off  OutDataTypeStr=boolean
  NOT1 : Logic  Operator=NOT  AllPortsSameDT=off  OutDataTypeStr=boolean
  Relational Operator1 : RelationalOperator  Operator=>  OutDataTypeStr=boolean  RndMeth=Simplest
  Switch2 : Switch  Criteria=u2 ~= 0
  Switch8 : Switch  Criteria=u2 ~= 0
  Switch9 : Switch  Criteria=u2 ~= 0
  Terminator : Terminator
  Test Detection Criteria1 : hcu_lib/Basic_Blocks/Test Detection Criteria
  Timer2 : hcu_lib/Basic_Blocks/Timer
  Unit Delay1 : UnitDelay  SampleTime=-1  HasFrameUpgradeWarning=on
  VDDM_C3CCU1CSDTC_raw32 : Outport
  VDDM_C3CCU1CSCFS_flg : Outport  Port=2
  wires:
  [DTC_clear_request] -> DTC_Info/4
  [VDDM_C3CCU1CSDet_flg] -> DTC_Info/1
  [VDDM_C3CCU1CSPass_flg] -> DTC_Info/2
  [VDDM_C3CCU1CSCFS_flg] -> DTC_Info/3
  DTC_Info/1 -> VDDM_C3CCU1CSDTC_raw32/1  "VDDM_C3CCU1CSDTC_raw32"
  DTC_clear_request/1 -> [DTC_clear_request]
  No_CAN3_BUS_OFF/1 -> [No_CAN3_BUS_OFF]
  task_time_s/1 -> [task_time_s]
  VDDM_C3CCU1CSChk_flg/1 -> [VDDM_C3CCU1CSChk_flg]
  VPMM_PwrStaSW_enum/1 -> [VPMM_PwrStaSW_enum]
  VPMM_PowerSta_enum/1 -> [VPMM_PowerSta_enum]
  VDDM_C3CCU1LCCFS_flg/1 -> [VDDM_C3CCU1LCCFS_flg]
  [No_CAN3_BUS_OFF] -> Logical Operator11/1
  Constant10/1 -> Equal8/2
  Equal5/1 -> Logical Operator17/2
  Logical Operator11/1 -> Switch2/2
  Switch2/1 -> Switch9/3
  Constant9/1 -> Switch9/1
  [task_time_s] -> Test Detection Criteria1/2
  [VPMM_PowerSta_enum] -> Equal8/1
  NOT1/1 -> Logical Operator22/2
  Constant6/1 -> Switch8/3
  Constant30/1 -> Logical Operator14/4
  Logical Operator14/1 -> [VDDM_C3CCU1CSCFSRls_flg]  "VDDM_C3CCU1CSCFSRls_flg"
  Constant7/1 -> Equal6/2
  [VDDM_C3CCU1CSPass_flg] -> Logical Operator22/1
  [VDDM_C3CCU1LCCFS_flg] -> Logical Operator10/1
  [VDDM_C3CCU1CSChk_flg] -> Switch2/1
  Unit Delay1/1 -> Equal7/1
  Constant8/1 -> Test Detection Criteria1/3
  Equal1/1 -> Logical Operator11/2
  [VDDM_C3CCU1CSCFS_flg] -> Delay1/1
  Switch8/1 -> Timer2/2, Logical Operator20/1
  [DTC_clear_request] -> Logical Operator14/2
  [VDDM_C3CCU1CSCFSRls_flg] -> DTC_Couter1/2
  Equal8/1 -> Logical Operator16/2
  Delay1/1 -> NOT1/1
  Logical Operator22/1 -> Logical Operator14/3
  Constant11/1 -> Relational Operator1/2
  Constant13/1 -> Switch2/3
  Constant29/1 -> Equal5/2
  Logical Operator20/1 -> Timer2/1
  Logical Operator16/1 -> Logical Operator14/1
  Constant17/1 -> Test Detection Criteria1/4
  Constant1/1 -> DTC_Couter1/3
  Constant14/1 -> Timer2/4
  Relational Operator1/1 -> Terminator/1  "VDDM_C3CCU1CSDFS_flg"
  DTC_Couter1/2 -> Relational Operator1/1  "VDDM_C3CCU1CSDTC_cnt"
  Constant12/1 -> Equal1/2
  Test Detection Criteria1/1 -> [VDDM_C3CCU1CSDet_flg]  "VDDM_C3CCU1CSDet_flg"
  Equal7/1 -> Logical Operator16/1
  [VDDM_C3CCU1CSDet_flg] -> DTC_Couter1/1
  Equal6/1 -> [VDDM_C3CCU1CSPass_flg]  "VDDM_C3CCU1CSPass_flg"
  DTC_Couter1/1 -> [VDDM_C3CCU1CSCFS_flg]  "VDDM_C3CCU1CSCFS_flg"
  [VDDM_C3CCU1CSChk_flg] -> Switch8/1
  Logical Operator17/1 -> Switch8/2
  [No_CAN3_BUS_OFF] -> Logical Operator17/1
  [VDDM_C3CCU1LCCFS_flg] -> Logical Operator13/1
  Switch9/1 -> Test Detection Criteria1/1
  [VPMM_PwrStaSW_enum] -> Equal1/1
  Logical Operator10/1 -> Logical Operator11/3
  [VPMM_PwrStaSW_enum] -> Equal5/1
  [task_time_s] -> Timer2/3
  [VDDM_C3CCU1CSCFSRls_flg] -> Switch9/2
  Constant31/1 -> Equal7/2
  Logical Operator13/1 -> Logical Operator17/3
  Timer2/1 -> Equal6/1
  [VPMM_PowerSta_enum] -> Unit Delay1/1
  [VDDM_C3CCU1CSCFS_flg] -> VDDM_C3CCU1CSCFS_flg/1

== system ddm/DDM/DDM/PMM/Comm err/The CAN signal between VCU and CCU2 is discontinuous ==
  note: Test Detection Criteria
  note: Release Condition After Decision
  note: Diagnostics and Fault Handling
  note: Test Pass Criteria
  task_time_s : Inport
  VPMM_PowerSta_enum : Inport  Port=2
  VPMM_PwrStaSW_enum : Inport  Port=3
  VDDM_C3CCU2RCChk_flg : Inport  Port=4
  VDDM_C3CCU2LCCFS_flg : Inport  Port=5
  No_CAN3_BUS_OFF : Inport  Port=6
  DTC_clear_request : Inport  Port=7
  Constant1 : Constant  Value=TRUE
  Constant10 : Constant  Value=ENUM_POWERSTA_STANDBY
  Constant11 : Constant  Value=ZERO_INT
  Constant12 : Constant  Value=FALSE
  Constant13 : Constant  Value=KDDM_C3CCU2RCPassTO_s
  Constant29 : Constant  Value=ENUM_PWRSTASW_OFF
  Constant30 : Constant  Value=KDDM_CommErrDiagnosisOffSW_flg
  Constant31 : Constant  Value=ENUM_POWERSTA_OFF
  Constant32 : Constant  Value=KDDM_C3CCU2RCDTC_cnt
  Constant33 : Constant  Value=KDDM_C3CCU2RCDetTO_s
  Constant6 : Constant  Value=KDDM_C3CCU2RCPassTO_s
  Constant7 : Constant  Value=KDDM_C3CCU2RCDTC_cnt
  Constant8 : Constant  Value=FALSE
  Constant9 : Constant  Value=ENUM_PWRSTASW_OFF
  DTC_Couter1 : hcu_lib/Basic_Blocks/DTC_Couter
  DTC_Info : hcu_lib/Basic_Blocks/DTC_Info
  Delay1 : Delay  DelayLength=1
  Equal1 : RelationalOperator  Operator=~=  OutDataTypeStr=boolean  RndMeth=Simplest
  Equal5 : RelationalOperator  Operator=~=  OutDataTypeStr=boolean  RndMeth=Simplest
  Equal6 : RelationalOperator  OutDataTypeStr=boolean  RndMeth=Simplest
  Equal7 : RelationalOperator  Operator===  OutDataTypeStr=boolean  RndMeth=Simplest
  Equal8 : RelationalOperator  Operator===  OutDataTypeStr=boolean  RndMeth=Simplest
  Logical Operator10 : Logic  Operator=NOT  AllPortsSameDT=off  OutDataTypeStr=boolean
  Logical Operator11 : Logic  Inputs=3  AllPortsSameDT=off  OutDataTypeStr=boolean
  Logical Operator13 : Logic  Operator=NOT  AllPortsSameDT=off  OutDataTypeStr=boolean
  Logical Operator14 : Logic  Operator=OR  Inputs=4  AllPortsSameDT=off  OutDataTypeStr=boolean
  Logical Operator16 : Logic  AllPortsSameDT=off  OutDataTypeStr=boolean
  Logical Operator17 : Logic  Inputs=3  AllPortsSameDT=off  OutDataTypeStr=boolean
  Logical Operator20 : Logic  Operator=NOT  AllPortsSameDT=off  OutDataTypeStr=boolean
  Logical Operator22 : Logic  AllPortsSameDT=off  OutDataTypeStr=boolean
  NOT1 : Logic  Operator=NOT  AllPortsSameDT=off  OutDataTypeStr=boolean
  Relational Operator1 : RelationalOperator  Operator=>  OutDataTypeStr=boolean  RndMeth=Simplest
  Switch2 : Switch  Criteria=u2 ~= 0
  Switch8 : Switch  Criteria=u2 ~= 0
  Switch9 : Switch  Criteria=u2 ~= 0
  Terminator : Terminator
  Test Detection Criteria1 : hcu_lib/Basic_Blocks/Test Detection Criteria
  Timer2 : hcu_lib/Basic_Blocks/Timer
  Unit Delay1 : UnitDelay  SampleTime=-1  HasFrameUpgradeWarning=on
  VDDM_C3CCU2RCDTC_raw32 : Outport
  VDDM_C3CCU2RCCFS_flg : Outport  Port=2
  wires:
  [VDDM_C3CCU2RCCFS_flg] -> VDDM_C3CCU2RCCFS_flg/1
  [DTC_clear_request] -> DTC_Info/4
  [VDDM_C3CCU2RCDet_flg] -> DTC_Info/1
  [VDDM_C3CCU2RCPass_flg] -> DTC_Info/2
  [VDDM_C3CCU2RCCFS_flg] -> DTC_Info/3
  DTC_Info/1 -> VDDM_C3CCU2RCDTC_raw32/1  "VDDM_C3CCU2RCDTC_raw32"
  DTC_clear_request/1 -> [DTC_clear_request]
  No_CAN3_BUS_OFF/1 -> [No_CAN3_BUS_OFF]
  task_time_s/1 -> [task_time_s]
  VDDM_C3CCU2RCChk_flg/1 -> [VDDM_C3CCU2RCChk_flg]
  VPMM_PwrStaSW_enum/1 -> [VPMM_PwrStaSW_enum]
  VPMM_PowerSta_enum/1 -> [VPMM_PowerSta_enum]
  VDDM_C3CCU2LCCFS_flg/1 -> [VDDM_C3CCU2LCCFS_flg]
  Relational Operator1/1 -> Terminator/1  "VDDM_C3CCU2RCDFS_flg"
  [VDDM_C3CCU2RCChk_flg] -> Switch2/1
  [VDDM_C3CCU2RCPass_flg] -> Logical Operator22/1
  [VDDM_C3CCU2RCCFSRls_flg] -> Switch9/2
  Equal6/1 -> [VDDM_C3CCU2RCPass_flg]  "VDDM_C3CCU2RCPass_flg"
  [VDDM_C3CCU2RCCFSRls_flg] -> DTC_Couter1/2
  [VPMM_PwrStaSW_enum] -> Equal1/1
  Equal5/1 -> Logical Operator17/2
  Equal7/1 -> Logical Operator16/1
  [task_time_s] -> Test Detection Criteria1/2
  [VPMM_PowerSta_enum] -> Unit Delay1/1
  Constant1/1 -> Switch8/3
  [DTC_clear_request] -> Logical Operator14/2
  Switch2/1 -> Switch9/3
  Logical Operator22/1 -> Logical Operator14/3
  NOT1/1 -> Logical Operator22/2
  Logical Operator13/1 -> Logical Operator17/3
  Constant30/1 -> Logical Operator14/4
  [No_CAN3_BUS_OFF] -> Logical Operator11/1
  [VPMM_PowerSta_enum] -> Equal8/1
  Switch9/1 -> Test Detection Criteria1/1
  Constant10/1 -> Equal8/2
  Constant9/1 -> Equal1/2
  [task_time_s] -> Timer2/3
  Logical Operator16/1 -> Logical Operator14/1
  Delay1/1 -> NOT1/1
  Logical Operator20/1 -> Timer2/1
  [No_CAN3_BUS_OFF] -> Logical Operator17/1
  DTC_Couter1/2 -> Relational Operator1/1  "VDDM_C3CCU2RCDTC_cnt"
  Constant31/1 -> Equal7/2
  Constant6/1 -> Equal6/2
  Constant12/1 -> Switch2/3
  Equal1/1 -> Logical Operator11/2
  Equal8/1 -> Logical Operator16/2
  Timer2/1 -> Equal6/1
  Constant8/1 -> Switch9/1
  Logical Operator17/1 -> Switch8/2
  Logical Operator10/1 -> Logical Operator11/3
  Constant29/1 -> Equal5/2
  [VDDM_C3CCU2RCCFS_flg] -> Delay1/1
  Logical Operator14/1 -> [VDDM_C3CCU2RCCFSRls_flg]  "VDDM_C3CCU2RCCFSRls_flg"
  Constant11/1 -> Relational Operator1/2
  Test Detection Criteria1/1 -> [VDDM_C3CCU2RCDet_flg]  "VDDM_C3CCU2RCDet_flg"
  Constant33/1 -> Test Detection Criteria1/4
  Constant13/1 -> Timer2/4
  Switch8/1 -> Timer2/2, Logical Operator20/1
  DTC_Couter1/1 -> [VDDM_C3CCU2RCCFS_flg]  "VDDM_C3CCU2RCCFS_flg"
  Constant32/1 -> Test Detection Criteria1/3
  Constant7/1 -> DTC_Couter1/3
  Logical Operator11/1 -> Switch2/2
  [VDDM_C3CCU2LCCFS_flg] -> Logical Operator13/1
  [VDDM_C3CCU2LCCFS_flg] -> Logical Operator10/1
  [VPMM_PwrStaSW_enum] -> Equal5/1
  [VDDM_C3CCU2RCDet_flg] -> DTC_Couter1/1
  [VDDM_C3CCU2RCChk_flg] -> Switch8/1
  Unit Delay1/1 -> Equal7/1

== system ddm/DDM/DDM/PMM/Comm err/The CAN signal between VCU and CCU2 is incomplete ==
  note: Test Detection Criteria
  note: Diagnostics and Fault Handling
  note: Release Condition After Decision
  note: Test Pass Criteria
  task_time_s : Inport
  VPMM_PowerSta_enum : Inport  Port=2
  VPMM_PwrStaSW_enum : Inport  Port=3
  VDDM_C3CCU2CSChk_flg : Inport  Port=4
  VDDM_C3CCU2LCCFS_flg : Inport  Port=5
  No_CAN3_BUS_OFF : Inport  Port=6
  DTC_clear_request : Inport  Port=7
  Constant1 : Constant  Value=KDDM_C3CCU2CSDTC_cnt
  Constant10 : Constant  Value=ENUM_POWERSTA_STANDBY
  Constant11 : Constant  Value=ZERO_INT
  Constant12 : Constant  Value=ENUM_PWRSTASW_OFF
  Constant13 : Constant  Value=FALSE
  Constant14 : Constant  Value=KDDM_C3CCU2CSPassTO_s
  Constant17 : Constant  Value=KDDM_C3CCU2CSDetTO_s
  Constant29 : Constant  Value=ENUM_PWRSTASW_OFF
  Constant30 : Constant  Value=KDDM_CommErrDiagnosisOffSW_flg
  Constant31 : Constant  Value=ENUM_POWERSTA_OFF
  Constant6 : Constant  Value=TRUE
  Constant7 : Constant  Value=KDDM_C3CCU2CSPassTO_s
  Constant8 : Constant  Value=KDDM_C3CCU2CSDTC_cnt
  Constant9 : Constant  Value=FALSE
  DTC_Couter1 : hcu_lib/Basic_Blocks/DTC_Couter
  DTC_Info : hcu_lib/Basic_Blocks/DTC_Info
  Delay1 : Delay  DelayLength=1
  Equal1 : RelationalOperator  Operator=~=  OutDataTypeStr=boolean  RndMeth=Simplest
  Equal5 : RelationalOperator  Operator=~=  OutDataTypeStr=boolean  RndMeth=Simplest
  Equal6 : RelationalOperator  OutDataTypeStr=boolean  RndMeth=Simplest
  Equal7 : RelationalOperator  Operator===  OutDataTypeStr=boolean  RndMeth=Simplest
  Equal8 : RelationalOperator  Operator===  OutDataTypeStr=boolean  RndMeth=Simplest
  Logical Operator10 : Logic  Operator=NOT  AllPortsSameDT=off  OutDataTypeStr=boolean
  Logical Operator11 : Logic  Inputs=3  AllPortsSameDT=off  OutDataTypeStr=boolean
  Logical Operator13 : Logic  Operator=NOT  AllPortsSameDT=off  OutDataTypeStr=boolean
  Logical Operator14 : Logic  Operator=OR  Inputs=4  AllPortsSameDT=off  OutDataTypeStr=boolean
  Logical Operator16 : Logic  AllPortsSameDT=off  OutDataTypeStr=boolean
  Logical Operator17 : Logic  Inputs=3  AllPortsSameDT=off  OutDataTypeStr=boolean
  Logical Operator20 : Logic  Operator=NOT  AllPortsSameDT=off  OutDataTypeStr=boolean
  Logical Operator22 : Logic  AllPortsSameDT=off  OutDataTypeStr=boolean
  NOT1 : Logic  Operator=NOT  AllPortsSameDT=off  OutDataTypeStr=boolean
  Relational Operator1 : RelationalOperator  Operator=>  OutDataTypeStr=boolean  RndMeth=Simplest
  Switch2 : Switch  Criteria=u2 ~= 0
  Switch8 : Switch  Criteria=u2 ~= 0
  Switch9 : Switch  Criteria=u2 ~= 0
  Terminator : Terminator
  Test Detection Criteria1 : hcu_lib/Basic_Blocks/Test Detection Criteria
  Timer2 : hcu_lib/Basic_Blocks/Timer
  Unit Delay1 : UnitDelay  SampleTime=-1  HasFrameUpgradeWarning=on
  VDDM_C3CCU2CSDTC_raw32 : Outport
  VDDM_C3CCU2CSCFS_flg : Outport  Port=2
  wires:
  [VDDM_C3CCU2CSCFS_flg] -> VDDM_C3CCU2CSCFS_flg/1
  [DTC_clear_request] -> DTC_Info/4
  [VDDM_C3CCU2CSDet_flg] -> DTC_Info/1
  [VDDM_C3CCU2CSPass_flg] -> DTC_Info/2
  [VDDM_C3CCU2CSCFS_flg] -> DTC_Info/3
  DTC_Info/1 -> VDDM_C3CCU2CSDTC_raw32/1  "VDDM_C3CCU2CSDTC_raw32"
  DTC_clear_request/1 -> [DTC_clear_request]
  No_CAN3_BUS_OFF/1 -> [No_CAN3_BUS_OFF]
  VDDM_C3CCU2LCCFS_flg/1 -> [VDDM_C3CCU2LCCFS_flg]
  VPMM_PowerSta_enum/1 -> [VPMM_PowerSta_enum]
  VPMM_PwrStaSW_enum/1 -> [VPMM_PwrStaSW_enum]
  VDDM_C3CCU2CSChk_flg/1 -> [VDDM_C3CCU2CSChk_flg]
  task_time_s/1 -> [task_time_s]
  Constant1/1 -> DTC_Couter1/3
  Logical Operator16/1 -> Logical Operator14/1
  Constant29/1 -> Equal5/2
  Logical Operator22/1 -> Logical Operator14/3
  Constant11/1 -> Relational Operator1/2
  Test Detection Criteria1/1 -> [VDDM_C3CCU2CSDet_flg]  "VDDM_C3CCU2CSDet_flg"
  Logical Operator13/1 -> Logical Operator17/3
  Timer2/1 -> Equal6/1
  [VPMM_PowerSta_enum] -> Unit Delay1/1
  [VPMM_PwrStaSW_enum] -> Equal5/1
  Switch9/1 -> Test Detection Criteria1/1
  [VPMM_PwrStaSW_enum] -> Equal1/1
  Logical Operator20/1 -> Timer2/1
  DTC_Couter1/1 -> [VDDM_C3CCU2CSCFS_flg]  "VDDM_C3CCU2CSCFS_flg"
  [task_time_s] -> Timer2/3
  Equal7/1 -> Logical Operator16/1
  DTC_Couter1/2 -> Relational Operator1/1  "VDDM_C3CCU2CSDTC_cnt"
  [No_CAN3_BUS_OFF] -> Logical Operator17/1
  Logical Operator17/1 -> Switch8/2
  [VDDM_C3CCU2LCCFS_flg] -> Logical Operator13/1
  [VDDM_C3CCU2CSChk_flg] -> Switch2/1
  Switch8/1 -> Timer2/2, Logical Operator20/1
  Unit Delay1/1 -> Equal7/1
  Constant31/1 -> Equal7/2
  [VDDM_C3CCU2CSCFSRls_flg] -> Switch9/2
  Equal1/1 -> Logical Operator11/2
  Constant6/1 -> Switch8/3
  [VPMM_PowerSta_enum] -> Equal8/1
  Logical Operator10/1 -> Logical Operator11/3
  NOT1/1 -> Logical Operator22/2
  [task_time_s] -> Test Detection Criteria1/2
  Equal6/1 -> [VDDM_C3CCU2CSPass_flg]  "VDDM_C3CCU2CSPass_flg"
  Constant10/1 -> Equal8/2
  Equal5/1 -> Logical Operator17/2
  Constant9/1 -> Switch9/1
  Relational Operator1/1 -> Terminator/1  "VDDM_C3CCU2CSDFS_flg"
  Constant12/1 -> Equal1/2
  Switch2/1 -> Switch9/3
  Logical Operator11/1 -> Switch2/2
  [No_CAN3_BUS_OFF] -> Logical Operator11/1
  [VDDM_C3CCU2CSDet_flg] -> DTC_Couter1/1
  Constant17/1 -> Test Detection Criteria1/4
  [VDDM_C3CCU2CSCFS_flg] -> Delay1/1
  Constant14/1 -> Timer2/4
  [VDDM_C3CCU2LCCFS_flg] -> Logical Operator10/1
  Constant13/1 -> Switch2/3
  [VDDM_C3CCU2CSChk_flg] -> Switch8/1
  Constant7/1 -> Equal6/2
  [VDDM_C3CCU2CSPass_flg] -> Logical Operator22/1
  Constant30/1 -> Logical Operator14/4
  Constant8/1 -> Test Detection Criteria1/3
  [DTC_clear_request] -> Logical Operator14/2
  Equal8/1 -> Logical Operator16/2
  [VDDM_C3CCU2CSCFSRls_flg] -> DTC_Couter1/2
  Logical Operator14/1 -> [VDDM_C3CCU2CSCFSRls_flg]  "VDDM_C3CCU2CSCFSRls_flg"
  Delay1/1 -> NOT1/1
